simulink model "SimulinkFurutaControl"  (R2017a)
settings: Solver=ode4  StartTime=0.0  StopTime=1.5  FixedStep=0.002  RelTol=1e-3
values from neighbouring files (symbols this model uses):
  Bb = 0.0015    [furuta.m]
  Bp = 0.0005    [furuta.m]
  Izz = 3.3282e-05    [furuta.m]
  Jb = 5.7198e-05    [furuta.m]
  k = place(A,B,p)    [furuta.m]
  Lb = 0.085    [furuta.m]
  Lbcm = 0.085/2    (= 0.0425)    [furuta.m]
  Lpcm = L/2    (= 0.0645)    [Pendulosimple_Linealizacion.m]    (also in furuta.m)
  Mb = 0.095    [furuta.m]
  Mp = 0.024    [furuta.m]
libraries: vrlib x1
settings Model: Creator=lmass  LastModifiedBy=David
settings OptimizationCC: LifeSpan=inf
settings DebuggingCC: SFExecutionAtInitializationDiag=none
settings HardwareCC: ProdBitPerSizeT=32  ProdBitPerPtrDiffT=32  ProdWordSize=32  ProdHWDeviceType=Specified

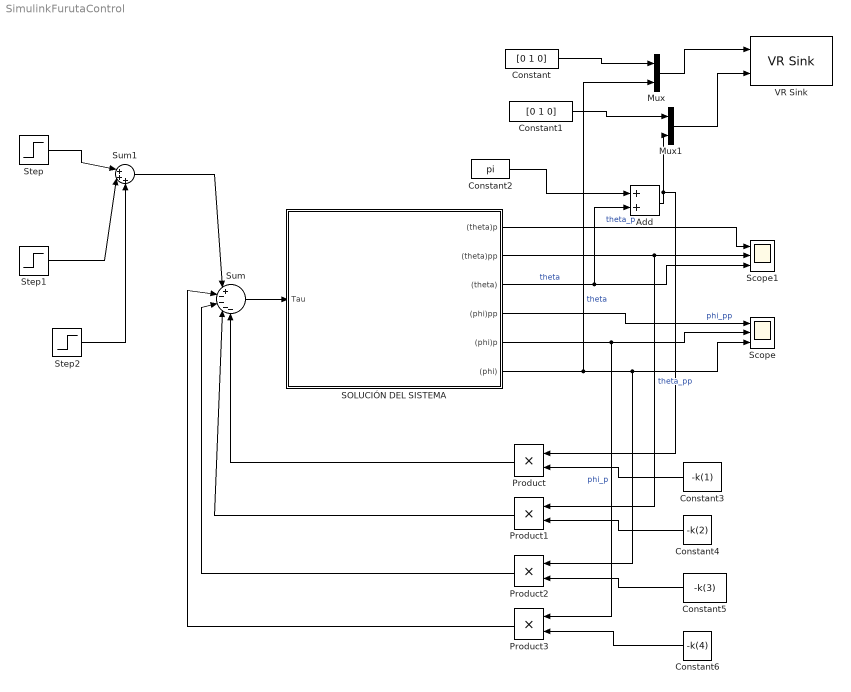
== system SimulinkFurutaControl ==
  Add : Sum
  Constant : Constant  Value=[0 1 0]
  Constant1 : Constant  Value=[0 1 0]
  Constant2 : Constant  Value=pi
  Constant3 : Constant  Value=-k(1)
  Constant4 : Constant  Value=-k(2)
  Constant5 : Constant  Value=-k(3)
  Constant6 : Constant  Value=-k(4)
  Mux : Mux  Inputs=2
  Mux1 : Mux  Inputs=2
  Product{,1..3} (4 alike) : Product
  SOLUCIÓN DEL SISTEMA : Subsystem
  Scope : Scope  NumInputPorts=3
  Scope1 : Scope  NumInputPorts=3
  Step : Step  After=0  SampleTime=0
  Step1 : Step  After=0  SampleTime=0
  Step2 : Step  After=0  SampleTime=0
  Sum : Sum  Inputs=|+----
  Sum1 : Sum  Inputs=|+++
  VR Sink : vrlib/VR Sink  InstantiateOnLoad=on  SampleTime=-1  ViewEnable=on  RemoteChange=off  RemoteView=off  FieldsWritten=Phi.rotation.4.1.1.double#Theta.rotation.4.1.1.double  WorldFileName=FurutaAnimacion.WRL  AutoView=off  VideoDimensions=[]  AllowVariableSize=off
      settings: SourceProductBaseCode=VR
  wires:
  SOLUCIÓN DEL SISTEMA/1((theta)p) -> Scope1/1  "theta_p"
  SOLUCIÓN DEL SISTEMA/2((theta)pp) -> Product1/1, Scope1/2  "theta_pp"
  SOLUCIÓN DEL SISTEMA/3((theta)) -> Add/2, Scope1/3  "theta"
  SOLUCIÓN DEL SISTEMA/4("(phi)pp ") -> Scope/1  "phi_pp"
  SOLUCIÓN DEL SISTEMA/5((phi)p) -> Product3/1, Scope/2  "phi_p"
  Constant/1 -> Mux/1
  Constant1/1 -> Mux1/1
  SOLUCIÓN DEL SISTEMA/6((phi)) -> Mux/2, Product2/1, Scope/3  "theta"
  Mux/1 -> VR Sink/1
  Mux1/1 -> VR Sink/2
  Add/1 -> Product/1, Mux1/2
  Constant2/1 -> Add/1
  Constant3/1 -> Product/2
  Constant4/1 -> Product1/2
  Constant5/1 -> Product2/2
  Constant6/1 -> Product3/2
  Sum/1 -> SOLUCIÓN DEL SISTEMA/1(Tau)
  Product/1 -> Sum/5
  Product1/1 -> Sum/4
  Product2/1 -> Sum/3
  Product3/1 -> Sum/2
  Step1/1 -> Sum1/2
  Step/1 -> Sum1/1
  Sum1/1 -> Sum/1
  Step2/1 -> Sum1/3

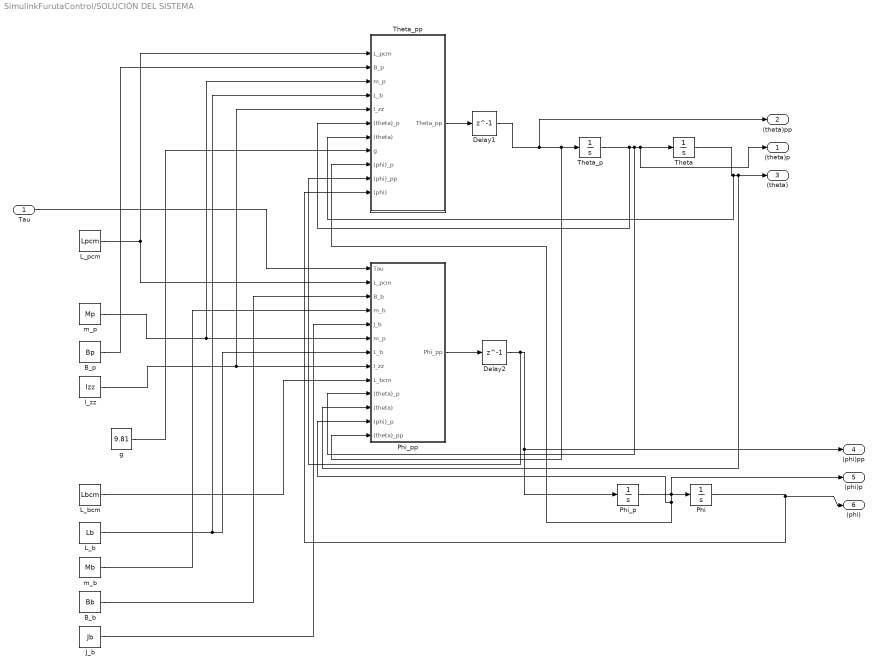
== system SimulinkFurutaControl/SOLUCIÓN DEL SISTEMA ==
  Tau : Inport
  B_b : Constant  Value=Bb
  B_p : Constant  Value=Bp
  Delay1 : Delay  DelayLength=1  InitialCondition=0  SampleTime=0.002
  Delay2 : Delay  DelayLength=1  InitialCondition=0  SampleTime=0.002
  I_zz : Constant  Value=Izz
  J_b : Constant  Value=Jb
  L_b : Constant  Value=Lb
  L_bcm : Constant  Value=Lbcm
  L_pcm : Constant  Value=Lpcm
  Phi : Integrator
  Phi_p : Integrator
  Phi_pp : Subsystem
  Theta : Integrator  InitialCondition=pi
  Theta_p : Integrator
  Theta_pp : Subsystem
  g : Constant  Value=9.81
  m_b : Constant  Value=Mb
  m_p : Constant  Value=Mp
  (theta)p : Outport
  (theta)pp : Outport  Port=2
  (theta) : Outport  Port=3
  "(phi)pp " : Outport  Port=4
  (phi)p : Outport  Port=5
  (phi) : Outport  Port=6
  wires:
  Theta_p/1 -> Theta_pp/6((theta)_p), Phi_pp/10((theta)_p), Theta/1, (theta)p/1
  Phi/1 -> (phi)/1, Theta_pp/11((phi))
  Tau/1 -> Phi_pp/1(Tau)
  L_pcm/1 -> Theta_pp/1(L_pcm), Phi_pp/2(L_pcm)
  B_b/1 -> Phi_pp/3(B_b)
  J_b/1 -> Phi_pp/5(J_b)
  m_p/1 -> Theta_pp/3(m_p), Phi_pp/6(m_p)
  L_b/1 -> Theta_pp/4("L_b "), Phi_pp/7("L_b ")
  I_zz/1 -> Theta_pp/5(I_zz), Phi_pp/8(I_zz)
  L_bcm/1 -> Phi_pp/9(L_bcm)
  g/1 -> Theta_pp/8(g)
  B_p/1 -> Theta_pp/2(B_p)
  m_b/1 -> Phi_pp/4(m_b)
  Phi_p/1 -> Phi/1, Phi_pp/12((phi)_p), Theta_pp/9((phi)_p), (phi)p/1
  Theta/1 -> Theta_pp/7((theta)), Phi_pp/11((theta)), (theta)/1
  Theta_pp/1(Theta_pp) -> Delay1/1
  Phi_pp/1(Phi_pp) -> Delay2/1
  Delay1/1 -> (theta)pp/1, Theta_p/1, Phi_pp/13(" (theta)_pp")
  Delay2/1 -> Theta_pp/10((phi)_pp), Phi_p/1, "(phi)pp "/1

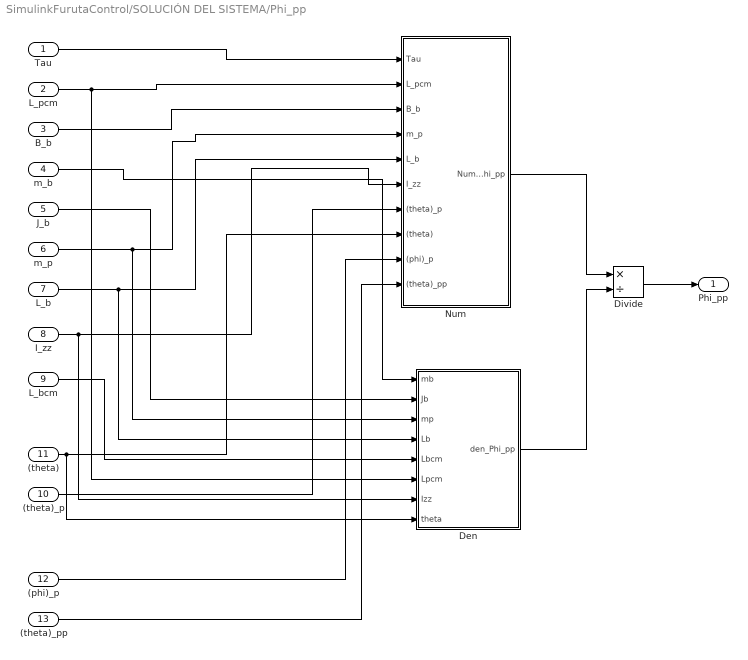
== system SimulinkFurutaControl/SOLUCIÓN DEL SISTEMA/Phi_pp ==
  Tau : Inport
  L_pcm : Inport  Port=2
  B_b : Inport  Port=3
  m_b : Inport  Port=4
  J_b : Inport  Port=5
  m_p : Inport  Port=6
  "L_b " : Inport  Port=7
  I_zz : Inport  Port=8
  L_bcm : Inport  Port=9
  (theta)_p : Inport  Port=10
  (theta) : Inport  Port=11
  (phi)_p : Inport  Port=12
  " (theta)_pp" : Inport  Port=13
  Den : Subsystem
  Divide : Product  Inputs=*/
  Num : Subsystem
  Phi_pp : Outport
  wires:
  Num/1(Num_Phi_pp) -> Divide/1
  Divide/1 -> Phi_pp/1
  Tau/1 -> Num/1(Tau)
  L_bcm/1 -> Den/5(Lbcm)
  I_zz/1 -> Den/7(Izz), Num/6(I_zz)
  "L_b "/1 -> Den/4(Lb), Num/5("L_b ")
  L_pcm/1 -> Den/6(Lpcm), Num/2(L_pcm)
  B_b/1 -> Num/3(B_b)
  m_b/1 -> Den/1(mb)
  J_b/1 -> Den/2("Jb ")
  m_p/1 -> Den/3(mp), Num/4(m_p)
  (theta)_p/1 -> Num/7((theta)_p)
  " (theta)_pp"/1 -> Num/10((theta)_pp)
  (phi)_p/1 -> Num/9((phi)_p)
  (theta)/1 -> Den/8(theta), Num/8((theta))
  Den/1("den_Phi_pp ") -> Divide/2

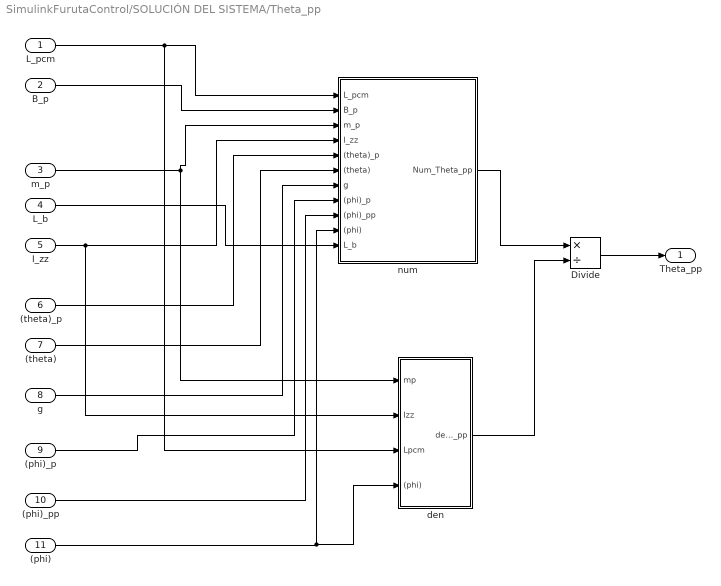
== system SimulinkFurutaControl/SOLUCIÓN DEL SISTEMA/Theta_pp ==
  L_pcm : Inport
  B_p : Inport  Port=2
  m_p : Inport  Port=3
  "L_b " : Inport  Port=4
  I_zz : Inport  Port=5
  (theta)_p : Inport  Port=6
  (theta) : Inport  Port=7
  g : Inport  Port=8
  (phi)_p : Inport  Port=9
  (phi)_pp : Inport  Port=10
  (phi) : Inport  Port=11
  Divide : Product  Inputs=*/
  den : Subsystem
  num : Subsystem
  Theta_pp : Outport
  wires:
  L_pcm/1 -> den/3(Lpcm), num/1(L_pcm)
  B_p/1 -> num/2(B_p)
  m_p/1 -> num/3(m_p), den/1(mp)
  I_zz/1 -> den/2("Izz "), num/4(I_zz)
  (theta)_p/1 -> num/5((theta)_p)
  g/1 -> num/7(g)
  num/1(Num_Theta_pp) -> Divide/1
  Divide/1 -> Theta_pp/1
  (phi)_pp/1 -> num/9((phi)_pp)
  (phi)_p/1 -> num/8((phi)_p)
  (phi)/1 -> den/4((phi)), num/10((phi))
  (theta)/1 -> num/6((theta))
  den/1("den_Theta_pp ") -> Divide/2
  "L_b "/1 -> num/11(L_b)

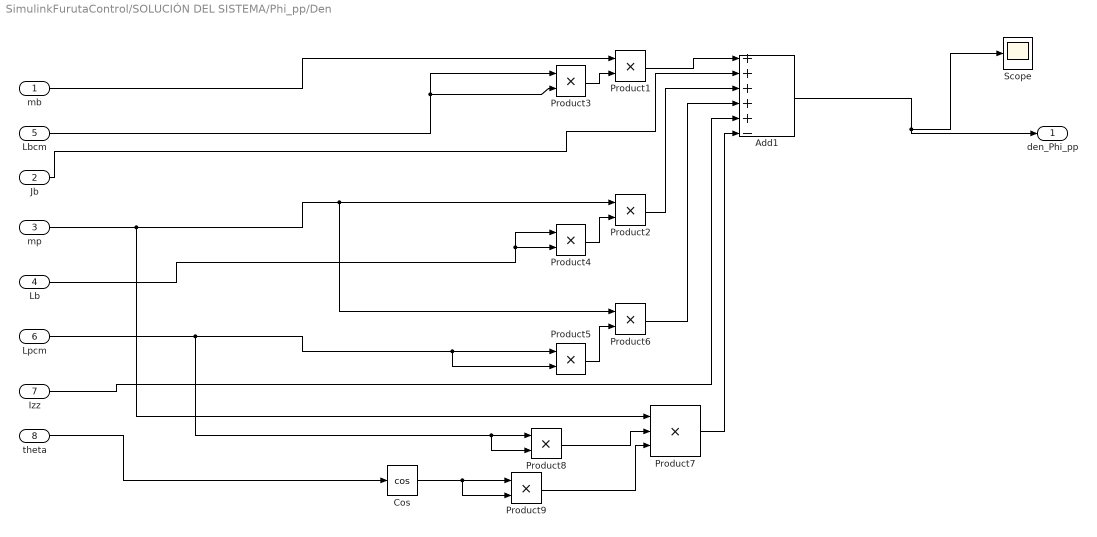
== system SimulinkFurutaControl/SOLUCIÓN DEL SISTEMA/Phi_pp/Den ==
  mb : Inport
  "Jb " : Inport  Port=2
  mp : Inport  Port=3
  Lb : Inport  Port=4
  Lbcm : Inport  Port=5
  Lpcm : Inport  Port=6
  Izz : Inport  Port=7
  theta : Inport  Port=8
  Add1 : Sum  Inputs=+++++-
  Cos : Trigonometry  Operator=cos
  Product{1..6,8..9} (8 alike) : Product
  Product7 : Product  Inputs=3
  Scope : Scope
  "den_Phi_pp " : Outport
  wires:
  Product4/1 -> Product2/2
  Product2/1 -> Add1/3
  Product8/1 -> Product7/2
  Product9/1 -> Product7/3
  Product3/1 -> Product1/2
  Product7/1 -> Add1/6
  Product1/1 -> Add1/1
  Product6/1 -> Add1/4
  Product5/1 -> Product6/2
  mb/1 -> Product1/1
  Lbcm/1 -> Product3/2, Product3/1
  "Jb "/1 -> Add1/2
  mp/1 -> Product7/1, Product6/1, Product2/1
  Lb/1 -> Product4/1, Product4/2
  Lpcm/1 -> Product8/2, Product8/1, Product5/2, Product5/1
  Izz/1 -> Add1/5
  Cos/1 -> Product9/2, Product9/1
  theta/1 -> Cos/1
  Add1/1 -> Scope/1, "den_Phi_pp "/1

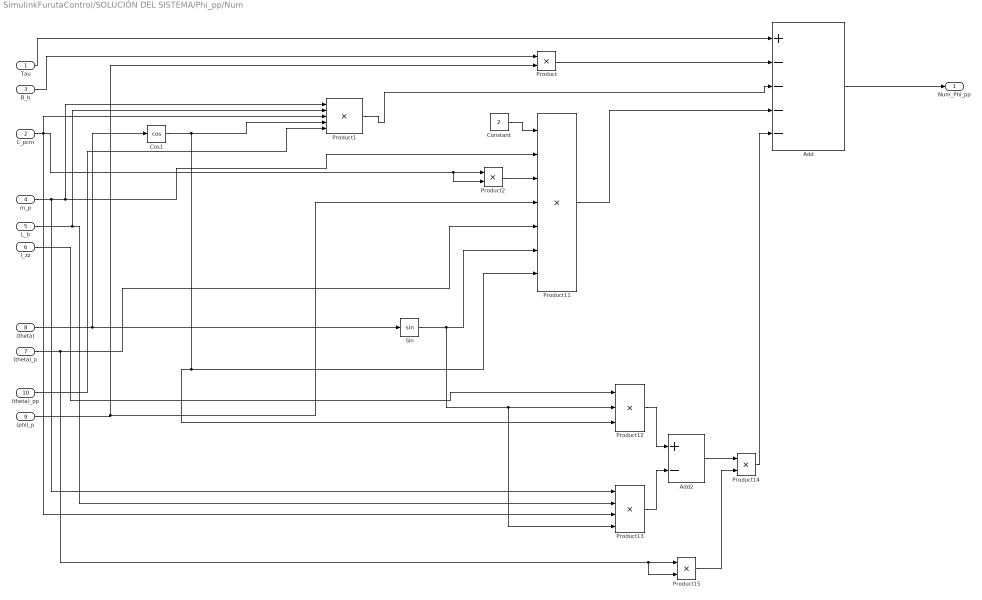
== system SimulinkFurutaControl/SOLUCIÓN DEL SISTEMA/Phi_pp/Num ==
  Tau : Inport
  L_pcm : Inport  Port=2
  B_b : Inport  Port=3
  m_p : Inport  Port=4
  "L_b " : Inport  Port=5
  I_zz : Inport  Port=6
  (theta)_p : Inport  Port=7
  (theta) : Inport  Port=8
  (phi)_p : Inport  Port=9
  (theta)_pp : Inport  Port=10
  Add : Sum  Inputs=+----
  Add2 : Sum  Inputs=+-
  Constant : Constant  Value=2
  Cos1 : Trigonometry  Operator=cos
  Product{,2,14..15} (4 alike) : Product
  Product1 : Product  Inputs=5
  Product11 : Product  Inputs=7
  Product12 : Product  Inputs=3
  Product13 : Product  Inputs=4
  Sin : Trigonometry
  Num_Phi_pp : Outport
  wires:
  Tau/1 -> Add/1
  B_b/1 -> Product/1
  (theta)_p/1 -> Product15/2, Product15/1, Product11/5
  Product/1 -> Add/2
  "L_b "/1 -> Product1/2, Product13/2
  m_p/1 -> Product13/1, Product1/1, Product11/2
  L_pcm/1 -> Product2/2, Product2/1, Product1/3, Product13/3
  I_zz/1 -> Product12/1
  Cos1/1 -> Product12/3, Product11/7, Product1/4
  (theta)/1 -> Cos1/1, Sin/1
  Product11/1 -> Add/4
  Constant/1 -> Product11/1
  (theta)_pp/1 -> Product1/5
  Sin/1 -> Product13/4, Product12/2, Product11/6
  Product12/1 -> Add2/1
  Product13/1 -> Add2/2
  Add2/1 -> Product14/1
  Product15/1 -> Product14/2
  Product14/1 -> Add/5
  Add/1 -> Num_Phi_pp/1
  Product1/1 -> Add/3
  (phi)_p/1 -> Product11/4, Product/2
  Product2/1 -> Product11/3

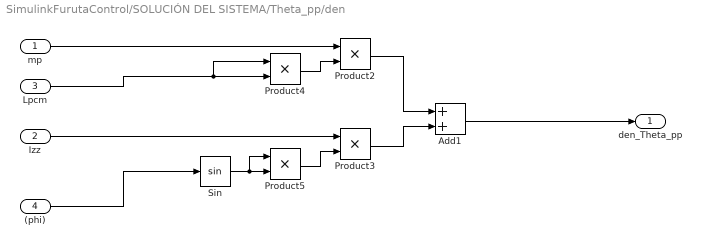
== system SimulinkFurutaControl/SOLUCIÓN DEL SISTEMA/Theta_pp/den ==
  mp : Inport
  "Izz " : Inport  Port=2
  Lpcm : Inport  Port=3
  (phi) : Inport  Port=4
  Add1 : Sum
  Product{2..5} (4 alike) : Product
  Sin : Trigonometry
  "den_Theta_pp " : Outport
  wires:
  Product5/1 -> Product3/2
  Product3/1 -> Add1/2
  Sin/1 -> Product5/1, Product5/2
  Product2/1 -> Add1/1
  Product4/1 -> Product2/2
  mp/1 -> Product2/1
  Lpcm/1 -> Product4/1, Product4/2
  "Izz "/1 -> Product3/1
  (phi)/1 -> Sin/1
  Add1/1 -> "den_Theta_pp "/1

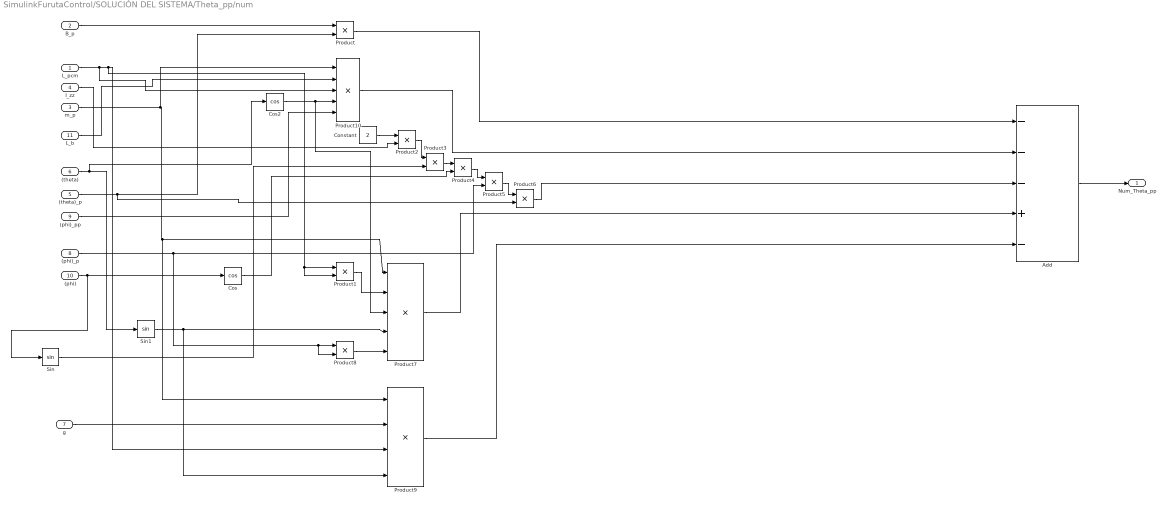
== system SimulinkFurutaControl/SOLUCIÓN DEL SISTEMA/Theta_pp/num ==
  L_pcm : Inport
  B_p : Inport  Port=2
  m_p : Inport  Port=3
  I_zz : Inport  Port=4
  (theta)_p : Inport  Port=5
  (theta) : Inport  Port=6
  g : Inport  Port=7
  (phi)_p : Inport  Port=8
  (phi)_pp : Inport  Port=9
  (phi) : Inport  Port=10
  L_b : Inport  Port=11
  Add : Sum  Inputs=---+-
  Constant : Constant  Value=2
  Cos : Trigonometry  Operator=cos
  Cos2 : Trigonometry  Operator=cos
  Product{,1..6,8} (8 alike) : Product
  Product10 : Product  Inputs=5
  Product7 : Product  Inputs=5
  Product9 : Product  Inputs=4
  Sin : Trigonometry
  Sin1 : Trigonometry
  Num_Theta_pp : Outport
  wires:
  Add/1 -> Num_Theta_pp/1
  B_p/1 -> Product/1
  (theta)_p/1 -> Product6/2, Product/2
  Product/1 -> Add/1
  m_p/1 -> Product10/1, Product9/1, Product7/1
  L_pcm/1 -> Product10/3, Product1/2, Product1/1, Product9/3
  I_zz/1 -> Product2/2
  (phi)/1 -> Sin/1, Cos/1
  Product6/1 -> Add/3
  Constant/1 -> Product2/1
  Cos/1 -> Product4/2
  (phi)_p/1 -> Product5/2, Product8/2, Product8/1
  Product7/1 -> Add/4
  Cos2/1 -> Product7/3, Product10/4
  Sin1/1 -> Product9/4, Product7/4
  Product8/1 -> Product7/5
  Product9/1 -> Add/5
  g/1 -> Product9/2
  (theta)/1 -> Cos2/1, Sin1/1
  Product10/1 -> Add/2
  L_b/1 -> Product10/2
  (phi)_pp/1 -> Product10/5
  Sin/1 -> Product3/2
  Product1/1 -> Product7/2
  Product2/1 -> Product3/1
  Product3/1 -> Product4/1
  Product4/1 -> Product5/1
  Product5/1 -> Product6/1
